simulink model "TestUSB_Rx"  (Simulink 6.4)
settings: Solver=FixedStepDiscrete  SolverMode=SingleTasking  StartTime=0  StopTime=inf  FixedStep=0.001  RelTol=1e-3
libraries: ecrobot_nxt_lib x8
CloseFcn:
  | rtwprivate ssgencode ModelCloseRequest TestBluetooth
settings Model: Creator=tchikama  LastModifiedBy=tchikama  ProdHWDeviceType=ARM7
settings DataIOCC: SaveOutput=off  SignalLogging=off  SaveTime=off
settings OptimizationCC: InlineParams=on  InlineInvariantSignals=on  RollThreshold=2  StateBitsets=on  DataBitsets=on  UseTempVars=on  InitFltsAndDblsToZero=off  NoFixptDivByZeroProtection=on  EfficientFloat2IntCast=on  OptimizeModelRefInitCode=on  LifeSpan=1
settings DebuggingCC: ConsistencyChecking=warning  SignalInfNanChecking=warning  ReadBeforeWriteMsg=DisableAll  WriteAfterWriteMsg=DisableAll  WriteAfterReadMsg=DisableAll  AlgebraicLoopMsg=error  CheckExecutionContextPreStartOutputMsg=on  CheckExecutionContextRuntimeOutputMsg=on  SolverPrmCheckMsg=none  SingleTaskRateTransMsg=warning  TasksWithSamePriorityMsg=none  IntegerOverflowMsg=error  ParameterPrecisionLossMsg=none  UnconnectedInputMsg=error  UnconnectedOutputMsg=error  UnconnectedLineMsg=error  UniqueDataStoreMsg=error  BusObjectLabelMismatch=error  RootOutportRequireBusObject=error  ModelReferenceIOMsg=warning  ModelReferenceVersionMismatchMessage=warning  ModelReferenceIOMismatchMessage=warning
settings HardwareCC: ProdIntDivRoundTo=Zero  ProdEndianess=LittleEndian  ProdHWDeviceType=ARM7  TargetHWDeviceType=32-bit Generic
settings ModelReferenceCC: ModelReferenceNumInstancesAllowed=Single
settings RTWCC: SystemTargetFile=ert.tlc  GenCodeOnly=on  GenerateMakefile=off  TemplateMakefile=ert_default_tmf  Description=Real-Time Workshop Embedded Coder (no auto configuration)  GenerateReport=on  RTWVerbose=off  ProcessScript=ert_make_rtw_hook  IncludeHyperlinkInReport=on  LaunchReport=on
settings CodeAppCC: ForceParamTrailComments=on  IgnoreCustomStorageClasses=off  SFDataObjDesc=on  PrefixModelToSubsysFcnNames=off  CustomSymbolStrGlobalVar=rt$N$M  CustomSymbolStrType=$N$M  CustomSymbolStrFcn=$N$M$F  CustomSymbolStrMacro=$N$M  InsertBlockDesc=on
settings ERTTargetCC: TargetFcnLib=ansi_tfl_tmw.mat  GenFloatMathFcnCalls=GNU  IncludeMdlTerminateFcn=off  SuppressErrorStatus=on  IncludeERTFirstTime=on  SupportAbsoluteTime=off  SupportNonFinite=off  SupportComplex=off  PurelyIntegerCode=on  InlinedParameterPlacement=NonHierarchical  RootIOFormat=Structure reference  ERTCustomFileTemplate=example_file_process.tlc  InitialValueSource=Model

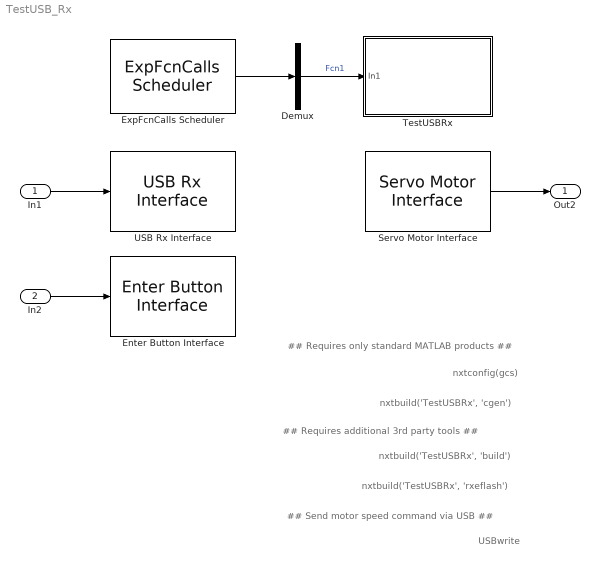
== system TestUSB_Rx ==
  note: nxtbuild('TestUSBRx', 'build')
  note: nxtbuild('TestUSBRx', 'rxeflash')
  note: nxtbuild('TestUSBRx', 'cgen')
  note: ## Requires only standard MATLAB products ##
  note: ## Requires additional 3rd party tools ##
  note: nxtconfig(gcs)
  note: ## Send motor speed command via USB ##
  note: USBwrite
  In1 : Inport
  In2 : Inport  Port=2
  Demux : Demux  Outputs=1
  Enter Button Interface : ecrobot_nxt_lib/Enter Button Interface  SystemSampleTime=-1
  ExpFcnCalls Scheduler : ecrobot_nxt_lib/ExpFcnCalls Scheduler  Priority=1  fcname='Fcn1'  fctrigger=[100]  ts=0.001  platform=OSEK  stacksize=[512]  bd_mode=Slave
  Servo Motor Interface : ecrobot_nxt_lib/Servo Motor Interface  SystemSampleTime=-1  ip=A  mode=Brake
  TestUSBRx : Subsystem
  USB Rx Interface : ecrobot_nxt_lib/USB Rx Interface  SystemSampleTime=-1
  Out2 : Outport
  wires:
  ExpFcnCalls Scheduler/1 -> Demux/1
  Demux/1 -> TestUSBRx/1(In1)  "Fcn1"
  Servo Motor Interface/1 -> Out2/1
  In1/1 -> USB Rx Interface/1
  In2/1 -> Enter Button Interface/1

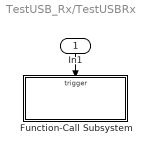
== system TestUSB_Rx/TestUSBRx ==
  In1 : Inport  Orientation=down
  Function-Call Subsystem : Subsystem  TreatAsAtomicUnit=on
  wires:
  In1/1 -> Function-Call Subsystem/Trigger

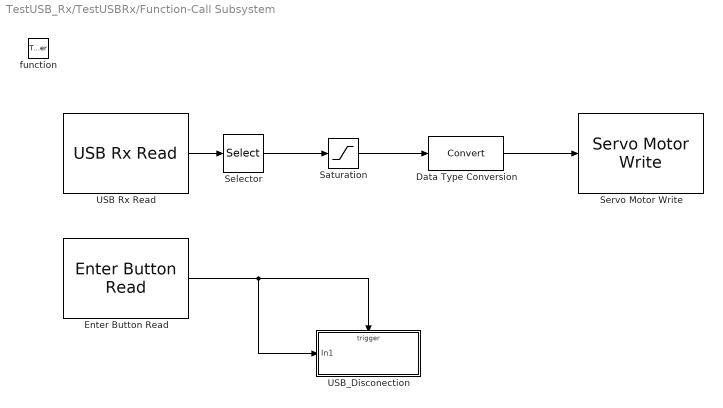
== system TestUSB_Rx/TestUSBRx/Function-Call Subsystem ==
  function : TriggerPort  TriggerType=function-call
  Data Type Conversion : DataTypeConversion
  Enter Button Read : ecrobot_nxt_lib/Enter Button Read  SystemSampleTime=-1
  Saturation : Saturate  UpperLimit=100  LowerLimit=0
  Selector : Selector  IndexMode=Zero-based  Elements=[0]  InputPortWidth=64
  Servo Motor Write : ecrobot_nxt_lib/Servo Motor Write  SystemSampleTime=-1  ip=A
  USB Rx Read : ecrobot_nxt_lib/USB Rx Read
  USB_Disconection : Subsystem  TreatAsAtomicUnit=on
  wires:
  USB Rx Read/1 -> Selector/1
  Selector/1 -> Saturation/1
  Saturation/1 -> Data Type Conversion/1
  Data Type Conversion/1 -> Servo Motor Write/1
  Enter Button Read/1 -> USB_Disconection/Trigger, USB_Disconection/1(In1)

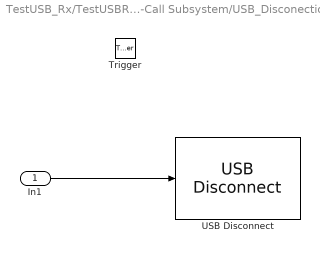
== system TestUSB_Rx/TestUSBRx/Function-Call Subsystem/USB_Disconection ==
  In1 : Inport
  Trigger : TriggerPort
  USB Disconnect : ecrobot_nxt_lib/USB Disconnect
  wires:
  In1/1 -> USB Disconnect/1
